simulink model "EISGov_Governor"  (R2016b)
settings: configuration reference "CodeGenConfigSet" (kept outside this file)
values from neighbouring files (symbols this model uses):
  EISGov_bEngSPDropRestrainEN_C = Calibration.Parameter    [init_EISGov_Governor.m]    (also in init_EISGov_Governor_SIL.m = Simulink.Parameter)
  EISGov_DKd_CUR = Calibration.Parameter    [init_EISGov_Governor.m]    (also in init_EISGov_Governor_SIL.m = Simulink.Parameter)
  EISGov_DKd_CURX = Calibration.Parameter    [init_EISGov_Governor.m]    (also in init_EISGov_Governor_SIL.m = Simulink.Parameter)
  EISGov_dnDiffHi_C = Calibration.Parameter    [init_EISGov_Governor.m]    (also in init_EISGov_Governor_SIL.m = Simulink.Parameter)
  EISGov_dnDiffLo_C = Calibration.Parameter    [init_EISGov_Governor.m]    (also in init_EISGov_Governor_SIL.m = Simulink.Parameter)
  EISGov_facDT1_CUR = Calibration.Parameter    [init_EISGov_Governor.m]    (also in init_EISGov_Governor_SIL.m = Simulink.Parameter)
  EISGov_facDT1_CURX = Calibration.Parameter    [init_EISGov_Governor.m]    (also in init_EISGov_Governor_SIL.m = Simulink.Parameter)
  EISGov_facPT1DiffLoFlt_C = Calibration.Parameter    [init_EISGov_Governor.m]    (also in init_EISGov_Governor_SIL.m = Simulink.Parameter)
  EISGov_facPT1TrqFlt_CUR = Calibration.Parameter    [init_EISGov_Governor.m]    (also in init_EISGov_Governor_SIL.m = Simulink.Parameter)
  EISGov_facPT1TrqFlt_CURX = Calibration.Parameter    [init_EISGov_Governor.m]    (also in init_EISGov_Governor_SIL.m = Simulink.Parameter)
  EISGov_nDHypDenom_C = Calibration.Parameter    [init_EISGov_Governor.m]    (also in init_EISGov_Governor_SIL.m = Simulink.Parameter)
  EISGov_nDHypNum_C = Calibration.Parameter    [init_EISGov_Governor.m]    (also in init_EISGov_Governor_SIL.m = Simulink.Parameter)
  EISGov_nDiffHi_C = Calibration.Parameter    [init_EISGov_Governor.m]    (also in init_EISGov_Governor_SIL.m = Simulink.Parameter)
  EISGov_nDiffHiLim_C = Calibration.Parameter    [init_EISGov_Governor.m]    (also in init_EISGov_Governor_SIL.m = Simulink.Parameter)
  EISGov_nDiffLo_C = Calibration.Parameter    [init_EISGov_Governor.m]    (also in init_EISGov_Governor_SIL.m = Simulink.Parameter)
  EISGov_stDTSlect_C = Calibration.Parameter    [init_EISGov_Governor.m]    (also in init_EISGov_Governor_SIL.m = Simulink.Parameter)
  EISGov_stIInitDemChange_C = Calibration.Parameter    [init_EISGov_Governor.m]    (also in init_EISGov_Governor_SIL.m = Simulink.Parameter)
  EISGov_swtTrqFltNeg_C = Calibration.Parameter    [init_EISGov_Governor.m]    (also in init_EISGov_Governor_SIL.m = Simulink.Parameter)
  EISGov_tiDT1_CUR = Calibration.Parameter    [init_EISGov_Governor.m]    (also in init_EISGov_Governor_SIL.m = Simulink.Parameter)
  EISGov_tiDT1_CURX = Calibration.Parameter    [init_EISGov_Governor.m]    (also in init_EISGov_Governor_SIL.m = Simulink.Parameter)
  EISGov_tiTimeSPDropResActive_CUR = Calibration.Parameter    [init_EISGov_Governor.m]    (also in init_EISGov_Governor_SIL.m = Simulink.Parameter)
  EISGov_tiTimeSPDropResActive_CURX = Calibration.Parameter    [init_EISGov_Governor.m]    (also in init_EISGov_Governor_SIL.m = Simulink.Parameter)
  EISGov_trqIHiLimMax_C = Calibration.Parameter    [init_EISGov_Governor.m]    (also in init_EISGov_Governor_SIL.m = Simulink.Parameter)
  EISGov_trqIHiLimMin_C = Calibration.Parameter    [init_EISGov_Governor.m]    (also in init_EISGov_Governor_SIL.m = Simulink.Parameter)
  EISGov_trqILoLimMax_C = Calibration.Parameter    [init_EISGov_Governor.m]    (also in init_EISGov_Governor_SIL.m = Simulink.Parameter)
  EISGov_trqILoLimMin_C = Calibration.Parameter    [init_EISGov_Governor.m]    (also in init_EISGov_Governor_SIL.m = Simulink.Parameter)
  EISGov_trqPIHiLimMax_C = Calibration.Parameter    [init_EISGov_Governor.m]    (also in init_EISGov_Governor_SIL.m = Simulink.Parameter)
  EISGov_trqPIHiLimMin_C = Calibration.Parameter    [init_EISGov_Governor.m]    (also in init_EISGov_Governor_SIL.m = Simulink.Parameter)
  EISGov_trqPILoLimMax_C = Calibration.Parameter    [init_EISGov_Governor.m]    (also in init_EISGov_Governor_SIL.m = Simulink.Parameter)
  EISGov_trqPILoLimMin_C = Calibration.Parameter    [init_EISGov_Governor.m]    (also in init_EISGov_Governor_SIL.m = Simulink.Parameter)
  LIGov_numTempSel_C = Calibration.Parameter    [init_EISGov_Governor.m]    (also in init_EISGov_Governor_SIL.m = Simulink.Parameter)
undefined symbols (not defined in the file or in its folder): EISGov_Governor_DT, EpmSynState_conv, HLSDem_KpCorFac_MAPX, I_S16, nseLib, Switch_conv
libraries: simulink x28, CXLib x15
(part 2 of 2)

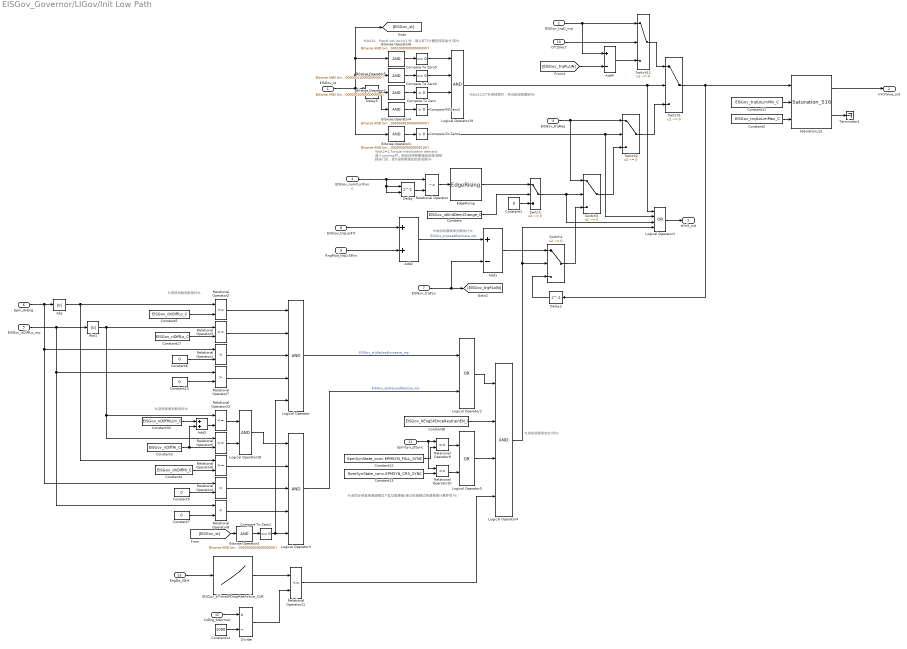
== system EISGov_Governor/LIGov/Init Low Path ==
  note: %全同步或者单曲轴模式下此功能使能(单凸轮轴模式转速梯度计算异常)%
  note: %发动机曲轴净负载估计%
  note: %突然卸载判断条件%
  note: %突然加载判断条件%
  note: %bit14，Prectl not lock=1 时，禁止DT1计算扭矩初始化I项%
  note: %突加突卸初始化I项%
  note: %bit11,DT补偿结束时，将当前扭矩赋给I%
  note: %bit2=1,Torque initialization demand
      | 进入running时，把启动扭矩赋值给怠速I扭矩
      | 踩油门后，把0扭矩赋值给怠速I扭矩%
  EISGov_st : Inport
  EISGov_trqD_mp : Inport  Port=2
  EISGov_trqReq : Inport  Port=3
  EISGov_numCurrFunc : Inport  Description=Identification name / number of the currently active EISGov client, which determines the current controller parameters  Port=4  OutDataTypeStr=Enum: EISGov_num_conv
  EISGov_nDiffLo_mp : Inport  Port=5
  Epm_dnEng : Inport  Tag=rpm/s  Description=Engine speed gradient calculated over current crankshaft-segment (S0-S0 or S1-S1)  Port=6  OutMin=-12000  OutMax=12000  OutDataTypeStr=EngSpeed_rpm_s
  EISGov_trqPLo : Inport  Port=7
  EISGov_trqLosFlt : Inport  Port=8
  RngMod_trqCrSMin : Inport  Port=9
  DT1Slect : Inport  Port=10
  EpmSyn_stSync : Inport  Port=11
  CoEng_tiNormal : Inport  Tag=ms  Description="Time since state\"CONENG_RUNNING\"was reached"  Port=12
  EngDa_tStrt : Inport  Description=state of starting system  Port=13
  Abs : Abs  SaturateOnIntegerOverflow=on
  Abs1 : Abs  OutDataTypeStr=Inherit: Inherit via back propagation
  Add1 : Sum  Inputs=+-  SaturateOnIntegerOverflow=on
  Add2 : Sum  SaturateOnIntegerOverflow=on
  Add3 : Sum
  Add4 : Sum  Inputs=+-  SaturateOnIntegerOverflow=on
  Bitwise Operator1 : simulink/Logic and Bit Operations/Bitwise Operator  logicop=AND  UseBitMask=on  BitMask=bin2dec('00000000000000000000000000000100')  BitMaskRealWorld=Stored Integer
  Bitwise Operator2 : simulink/Logic and Bit Operations/Bitwise Operator  logicop=AND  UseBitMask=on  BitMask=bin2dec('00000000000000000000100000000000')  BitMaskRealWorld=Stored Integer
  Bitwise Operator3 : simulink/Logic and Bit Operations/Bitwise Operator  logicop=AND  UseBitMask=on  BitMask=bin2dec('00000000000010000000000000000000')  BitMaskRealWorld=Stored Integer
  Bitwise Operator4 : simulink/Logic and Bit Operations/Bitwise Operator  logicop=AND  UseBitMask=on  BitMask=bin2dec('00000000000000000000010000000000')  BitMaskRealWorld=Stored Integer
  Bitwise Operator5 : simulink/Logic and Bit Operations/Bitwise Operator  logicop=AND  UseBitMask=on  BitMask=bin2dec('00000000000000000000110000000000')  BitMaskRealWorld=Stored Integer
  Bitwise Operator6 : simulink/Logic and Bit Operations/Bitwise Operator  logicop=AND  UseBitMask=on  BitMask=bin2dec('00000000000000000100000000000000')  BitMaskRealWorld=Stored Integer
  Compare To Zero : simulink/Logic and Bit Operations/Compare To Zero  relop=>  OutDataTypeStr=boolean
  Compare To Zero1 : simulink/Logic and Bit Operations/Compare To Zero  relop===  OutDataTypeStr=boolean
  Compare To Zero2 : simulink/Logic and Bit Operations/Compare To Zero  relop=>  OutDataTypeStr=boolean
  Compare To Zero3 : simulink/Logic and Bit Operations/Compare To Zero  relop===  OutDataTypeStr=boolean
  Compare To Zero4 : simulink/Logic and Bit Operations/Compare To Zero  relop=>  OutDataTypeStr=boolean
  Compare To Zero5 : simulink/Logic and Bit Operations/Compare To Zero  relop===  OutDataTypeStr=boolean
  Constant : Constant  Value=EISGov_stIInitDemChange_C
  Constant1 : Constant  Value=0  OutDataTypeStr=Inherit: Inherit via back propagation
  Constant{6..7,9..10} (4 alike) : Constant  Value=0  OutDataTypeStr=Inherit: Inherit via back propagation  SampleTime=-1
  Constant11 : Constant  Value=EISGov_trqILoLimMin_C
  Constant12 : Constant  Value=EpmSynState_conv.EPMSYN_FULL_SYNC
  Constant13 : Constant  Value=EpmSynState_conv.EPMSYN_CRS_SYNC
  Constant14 : Constant  Value=1000  OutDataTypeStr=Inherit: Inherit via back propagation
  Constant17 : Constant  Value=EISGov_nDiffLo_C  SampleTime=-1
  Constant2 : Constant  Value=EISGov_trqILoLimMax_C
  Constant3 : Constant  Value=EISGov_nDiffHi_C  SampleTime=-1
  Constant30 : Constant  Value=EISGov_nDiffHiLim_C  SampleTime=-1
  Constant4 : Constant  Value=EISGov_dnDiffHi_C  SampleTime=-1
  Constant5 : Constant  Value=EISGov_dnDiffLo_C  SampleTime=-1
  Constant8 : Constant  Value=EISGov_bEngSPDropRestrainEN_C  SampleTime=-1
  Delay : Delay  DelayLength=1  InitialConditionSource=Input port  InitialCondition=0
      settings: InputPortMap=u0,p4
  Delay2 : Delay  DelayLength=1  InitialCondition=0
  Delay5 : Delay  DelayLength=1  InitialConditionSource=Input port  InitialCondition=0
      settings: InputPortMap=u0,p4
  Divide : Product  Inputs=*/  OutDataTypeStr=Inherit: Inherit via back propagation
  EISGov_tiTimeSPDropResActive_CUR : Lookup_n-D  NumberOfTableDimensions=1  BreakpointsForDimension1=EISGov_tiTimeSPDropResActive_CURX  BreakpointsForDimension2=HLSDem_KpCorFac_MAPX  Table=EISGov_tiTimeSPDropResActive_CUR  ExtrapMethod=Clip  InternalRulePriority=Speed  OutDataTypeStr=Inherit: Inherit via back propagation  RndMeth=Simplest  SaturateOnIntegerOverflow=on
  EdgeRising : CXLib/EdgeRising
  Logical Operator : Logic  Inputs=5  AllPortsSameDT=off  OutDataTypeStr=boolean
  Logical Operator1 : Logic  Operator=OR  Inputs=4  AllPortsSameDT=off  OutDataTypeStr=boolean
  Logical Operator18 : Logic  AllPortsSameDT=off  OutDataTypeStr=boolean
  Logical Operator19 : Logic  Inputs=4  AllPortsSameDT=off  OutDataTypeStr=boolean
  Logical Operator2 : Logic  Operator=OR  AllPortsSameDT=off  OutDataTypeStr=boolean
  Logical Operator3 : Logic  Inputs=5  AllPortsSameDT=off  OutDataTypeStr=boolean
  Logical Operator4 : Logic  Inputs=4  AllPortsSameDT=off  OutDataTypeStr=boolean
  Logical Operator5 : Logic  Operator=OR  AllPortsSameDT=off  OutDataTypeStr=boolean
  Relational Operator : RelationalOperator  Operator=~=  OutDataTypeStr=boolean  RndMeth=Simplest
  Relational Operator1 : RelationalOperator  Operator=<  OutDataTypeStr=boolean  RndMeth=Nearest  InputSameDT=on
  Relational Operator10 : RelationalOperator  Operator===  OutDataTypeStr=boolean  RndMeth=Simplest
  Relational Operator11 : RelationalOperator  Operator=<=  OutDataTypeStr=boolean  RndMeth=Simplest  InputSameDT=on
  Relational Operator{2..3,5..6} (4 alike) : RelationalOperator  OutDataTypeStr=boolean  RndMeth=Nearest  InputSameDT=on
  Relational Operator23 : RelationalOperator  Operator=<=  OutDataTypeStr=boolean  RndMeth=Nearest  InputSameDT=on
  Relational Operator4 : RelationalOperator  Operator=>  OutDataTypeStr=boolean  RndMeth=Nearest  InputSameDT=on
  Relational Operator7 : RelationalOperator  Operator=>  OutDataTypeStr=boolean  RndMeth=Nearest  InputSameDT=on
  Relational Operator8 : RelationalOperator  Operator=<  OutDataTypeStr=boolean  RndMeth=Nearest  InputSameDT=on
  Relational Operator9 : RelationalOperator  Operator===  OutDataTypeStr=boolean  RndMeth=Simplest
  Saturation_S2 : CXLib/Saturation_S16
  Switch : Switch  Criteria=u2 ~= 0
  Switch{1..4} (4 alike) : Switch  Criteria=u2 ~= 0  InputSameDT=on
  Switch11 : Switch  Criteria=u2 ~= 0
  Terminator1 : Terminator
  stInit_out : Outport
  InitValue_out : Outport  Port=2
  wires:
  Logical Operator19/1 -> Logical Operator1/1, Switch1/2
  Bitwise Operator2/1 -> Compare To Zero/1
  Switch1/1 -> Delay2/1, Saturation_S2/1
  Bitwise Operator1/1 -> Compare To Zero4/1
  Switch2/1 -> Switch1/3
  Logical Operator1/1 -> stInit_out/1
  EISGov_st/1 -> Delay5/2, Bitwise Operator1/1, Delay5/1, [EISGov_st], Bitwise Operator6/1, Bitwise Operator5/1
  EISGov_trqReq/1 -> Switch3/1, Switch2/1
  Switch3/1 -> Switch2/3
  EISGov_numCurrFunc/1 -> Delay/1, Delay/2, Relational Operator/1
  Delay/1 -> Relational Operator/2
  Relational Operator/1 -> EdgeRising/1
  Switch/1 -> Logical Operator1/3, Switch3/2
  EdgeRising/1 -> Switch/1
  Constant/1 -> Switch/2
  Constant1/1 -> Switch/3
  Constant11/1 -> Saturation_S2/2
  Constant2/1 -> Saturation_S2/3
  Saturation_S2/1 -> InitValue_out/1
  Saturation_S2/2 -> Terminator1/1
  Relational Operator6/1 -> Logical Operator3/2
  Relational Operator3/1 -> Logical Operator/2
  Relational Operator2/1 -> Logical Operator/1
  Constant4/1 -> Relational Operator6/2
  Constant17/1 -> Relational Operator3/2
  Constant5/1 -> Relational Operator2/2
  Constant3/1 -> Add3/2, Relational Operator5/2
  Relational Operator1/1 -> Logical Operator/3
  Relational Operator4/1 -> Logical Operator3/3
  Logical Operator/1 -> Logical Operator2/1  "EISGov_stIdleLoadIncrease_mp"
  Logical Operator3/1 -> Logical Operator2/2  "EISGov_stIdleLoadReduce_mp"
  Switch4/1 -> Switch3/3
  Delay2/1 -> Switch4/3
  EISGov_trqLosFlt/1 -> Add2/1
  Constant6/1 -> Relational Operator1/2
  Constant7/1 -> Relational Operator8/2
  Relational Operator7/1 -> Logical Operator/4
  Bitwise Operator3/1 -> Compare To Zero1/1
  [EISGov_st] -> Bitwise Operator3/1
  Relational Operator8/1 -> Logical Operator3/4
  Compare To Zero1/1 -> Logical Operator/5, Logical Operator3/5
  Constant8/1 -> Logical Operator4/2
  Logical Operator2/1 -> Logical Operator4/1
  RngMod_trqCrSMin/1 -> Add2/2
  Constant9/1 -> Relational Operator4/2
  Constant10/1 -> Relational Operator7/2
  Abs1/1 -> Relational Operator3/1, Relational Operator23/1, Relational Operator5/1
  Logical Operator4/1 -> Logical Operator1/4, Switch4/2
  Add1/1 -> Switch4/1
  Add2/1 -> Add1/1  "EISGov_trqLoadEstimate_mp"
  EISGov_nDiffLo_mp/1 -> Relational Operator8/1, Relational Operator7/1, Abs1/1
  Epm_dnEng/1 -> Relational Operator4/1, Relational Operator1/1, Abs/1
  Abs/1 -> Relational Operator6/1, Relational Operator2/1
  Add3/1 -> Relational Operator23/2
  Constant30/1 -> Add3/1
  Relational Operator23/1 -> Logical Operator18/1
  Relational Operator5/1 -> Logical Operator18/2
  Logical Operator18/1 -> Logical Operator3/1
  EISGov_trqD_mp/1 -> Switch11/1, Add4/1
  [EISGov_trqPLoIN] -> Add4/2
  Add4/1 -> Switch11/3
  Switch11/1 -> Switch1/1
  DT1Slect/1 -> Switch11/2
  Bitwise Operator4/1 -> Compare To Zero2/1
  Bitwise Operator5/1 -> Compare To Zero3/1
  Delay5/1 -> Bitwise Operator4/1, Bitwise Operator2/1
  EISGov_trqPLo/1 -> Add1/2, [EISGov_trqPLoIN]
  Bitwise Operator6/1 -> Compare To Zero5/1
  Compare To Zero2/1 -> Logical Operator19/4
  Compare To Zero/1 -> Logical Operator19/3
  Compare To Zero3/1 -> Logical Operator19/2
  Compare To Zero5/1 -> Logical Operator19/1
  Compare To Zero4/1 -> Logical Operator1/2, Switch2/2
  EpmSyn_stSync/1 -> Relational Operator10/1, Relational Operator9/1
  Constant12/1 -> Relational Operator9/2
  Constant13/1 -> Relational Operator10/2
  Relational Operator9/1 -> Logical Operator5/1
  Relational Operator10/1 -> Logical Operator5/2
  Logical Operator5/1 -> Logical Operator4/3
  CoEng_tiNormal/1 -> Divide/1
  Constant14/1 -> Divide/2
  EISGov_tiTimeSPDropResActive_CUR/1 -> Relational Operator11/1
  Divide/1 -> Relational Operator11/2
  Relational Operator11/1 -> Logical Operator4/4
  EngDa_tStrt/1 -> EISGov_tiTimeSPDropResActive_CUR/1

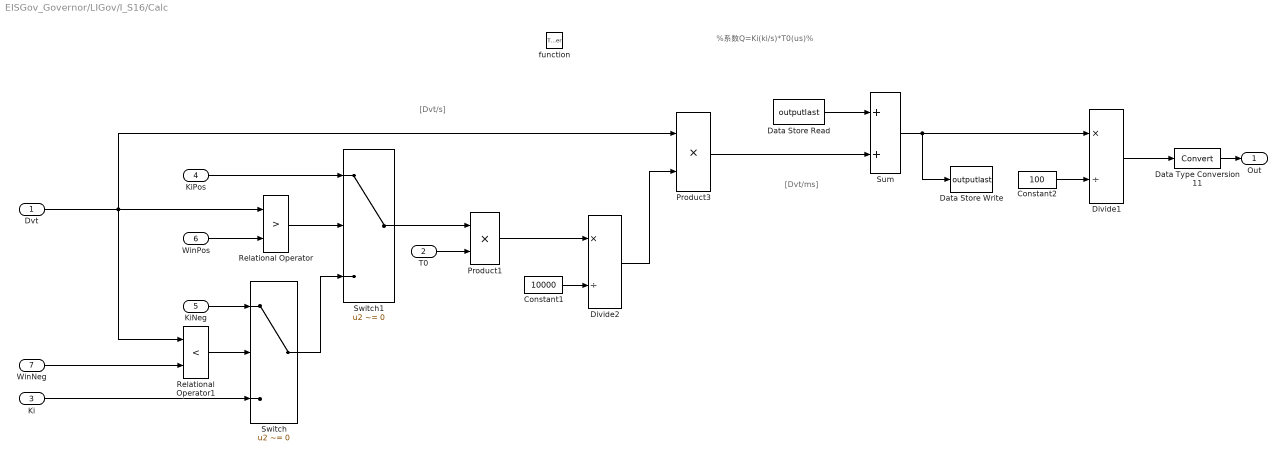
== system EISGov_Governor/LIGov/I_S16/Calc ==
  note: %系数Q=Ki(ki/s)*T0(us)%
  note: [Dvt/s]
  note: [Dvt/ms]
  Dvt : Inport
  T0 : Inport  Port=2
  Ki : Inport  Port=3
  KiPos : Inport  Port=4
  KiNeg : Inport  Port=5
  WinPos : Inport  Port=6
  WinNeg : Inport  Port=7
  function : TriggerPort  TriggerType=function-call  VariantControl=Variant
  Constant1 : Constant  Value=10000  OutDataTypeStr=uint32
  Constant2 : Constant  Value=100  OutDataTypeStr=uint32
  Data Store Read : DataStoreRead  DataStoreName=outputlast
  Data Store Write : DataStoreWrite  DataStoreName=outputlast
  Data Type Conversion11 : DataTypeConversion  SaturateOnIntegerOverflow=on
  Divide1 : Product  Inputs=*/  OutDataTypeStr=fixdt(1,32,0.00001,0)  RndMeth=Round  SaturateOnIntegerOverflow=on
  Divide2 : Product  Inputs=*/  OutDataTypeStr=fixdt(1,32,0.0001,0)  RndMeth=Round  SaturateOnIntegerOverflow=on
  Product1 : Product  OutDataTypeStr=fixdt(1,32,0.001,0)  RndMeth=Round  SaturateOnIntegerOverflow=on
  Product3 : Product  OutDataTypeStr=fixdt(1,32,0.001,0)  RndMeth=Round  SaturateOnIntegerOverflow=on
  Relational Operator : RelationalOperator  Operator=>  OutDataTypeStr=boolean  RndMeth=Nearest  InputSameDT=on
  Relational Operator1 : RelationalOperator  Operator=<  OutDataTypeStr=boolean  RndMeth=Nearest  InputSameDT=on
  Sum : Sum  OutDataTypeStr=Inherit: Inherit via back propagation  RndMeth=Round  SaturateOnIntegerOverflow=on  InputSameDT=on
  Switch : Switch  Criteria=u2 ~= 0  SaturateOnIntegerOverflow=on  InputSameDT=on
  Switch1 : Switch  Criteria=u2 ~= 0  SaturateOnIntegerOverflow=on  InputSameDT=on
  Out : Outport
  wires:
  Product3/1 -> Sum/2
  Divide1/1 -> Data Type Conversion11/1
  Divide2/1 -> Product3/2
  Constant1/1 -> Divide2/2
  Product1/1 -> Divide2/1
  Data Type Conversion11/1 -> Out/1
  Constant2/1 -> Divide1/2
  Sum/1 -> Data Store Write/1, Divide1/1
  Dvt/1 -> Relational Operator1/1, Relational Operator/1, Product3/1
  Switch1/1 -> Product1/1
  T0/1 -> Product1/2
  WinNeg/1 -> Relational Operator1/2
  Ki/1 -> Switch/3
  Data Store Read/1 -> Sum/1
  Switch/1 -> Switch1/3
  WinPos/1 -> Relational Operator/2
  Relational Operator1/1 -> Switch/2
  KiNeg/1 -> Switch/1
  Relational Operator/1 -> Switch1/2
  KiPos/1 -> Switch1/1

== system EISGov_Governor/LIGov/I_S16/Init ==
  InitVal : Inport
  function : TriggerPort  TriggerType=function-call  VariantControl=Variant
  Constant2 : Constant  Value=100  OutDataTypeStr=uint32
  Data Store Write : DataStoreWrite  DataStoreName=outputlast
  Divide1 : Product  Inputs=**  OutDataTypeStr=fixdt(1,32,0.001,0)  RndMeth=Round  SaturateOnIntegerOverflow=on
  wires:
  Constant2/1 -> Divide1/2
  Divide1/1 -> Data Store Write/1
  InitVal/1 -> Divide1/1

== stateflow chart EISGov_Governor/LIGov/I_S16/Chart ==
  (default) -> (junction 1)
  (junction 1) -> (junction 3) [order 2] : {CalcCal;}
  (junction 1) -> (junction 5) [order 1] : [stInit == 1]
      | {InitCal;}
  (junction 5) -> (junction 6)
  (junction 3) -> (junction 6)
  data: stInit input boolean
  events: InitCal output FUNCTION_CALL_EVENT; CalcCal output FUNCTION_CALL_EVENT
